simulink model "AthenaSim_2"  (R2024b)
settings: Solver=ode4  StartTime=0.0  StopTime=inf  FixedStep=0.001  RelTol=1e-3
undefined symbols (not defined in the file or in its folder): Payload
libraries: uavmavlinklib x4, dspnetwork x2, shared6dof x1
settings Model: Creator=ercu  LastModifiedBy=ercu

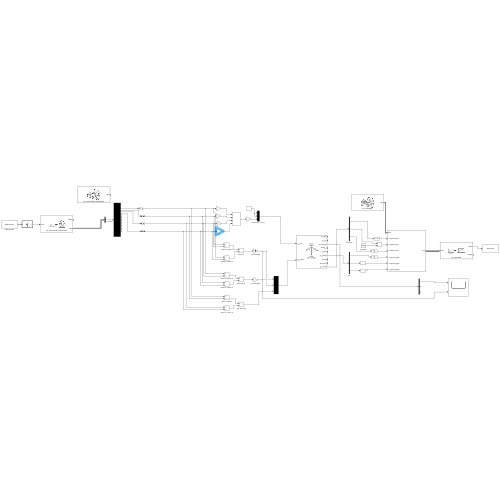
[thumbnail: Simulink's stored preview of the top-level diagram]
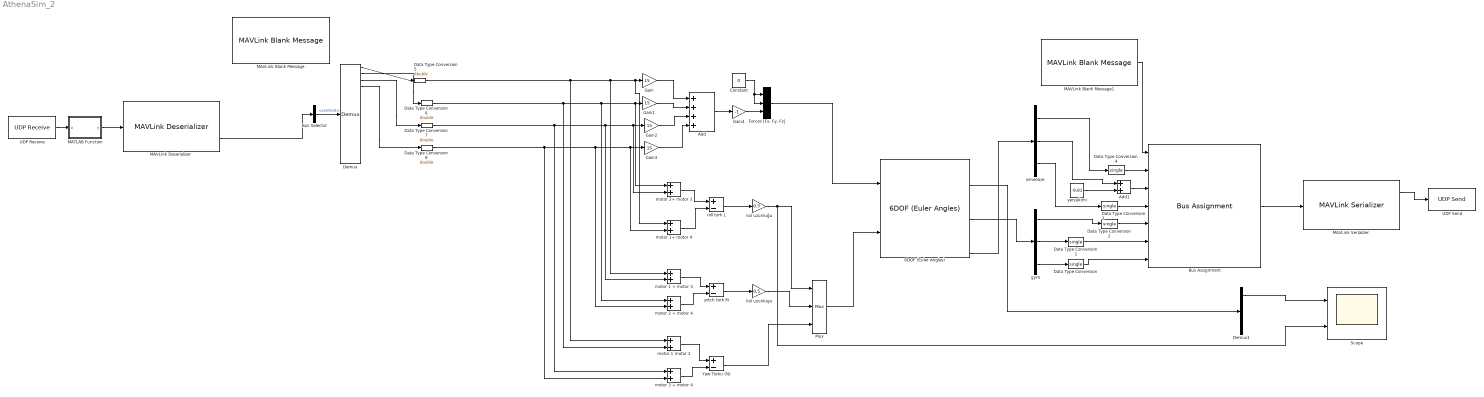
== system AthenaSim_2 ==
  6DOF (Euler Angles) : shared6dof/6DOF (Euler Angles)  units=Metric (MKS)  mtype=Fixed  rep=Euler Angles  xme_0=[0 0 0]  Vm_0=[0 0 0]  eul_0=[0.5 0 0]  pm_0=[0 0 0]  mass_0=1.0  mass_e=0.5  mass_f=2.0  inertia=eye(3) * 0.08  inertia_e=eye(3)  inertia_f=2*eye(3)  k_quat=1.0  vre_flag=on  abi_flag=on  aMode=0  xme_statename=''  Vm_statename=''  eul_statename=''  quat_statename=''  pm_statename=''  mass_statename=''
  Add : Sum  Inputs=++++  OutDataTypeStr=double
  Add1 : Sum  OutDataTypeStr=single
  Bus Assignment : BusAssignment  AssignedSignals=Payload.xacc,Payload.yacc,Payload.zacc,Payload.xgyro,Payload.ygyro,Payload.zgyro
  Bus Selector : BusSelector  OutputSignals=Payload.controls
  Constant : Constant  Value=0
  Data Type Conversion{,1..4} (5 alike) : DataTypeConversion  OutDataTypeStr=single  SaturateOnIntegerOverflow=off  RndMeth=Floor
  Data Type Conversion{5..8} (4 alike) : DataTypeConversion  OutDataTypeStr=double  SaturateOnIntegerOverflow=off  RndMeth=Floor
  Demux : Demux  Outputs=16
  Demux1 : Demux  Outputs=3
  "Forces [Fx, Fy, Fz]" : Mux  Inputs=3
  Gain{,1..3} (4 alike) : Gain  Gain=15
  Gain4 : Gain  Gain=-1
  MATLAB Function : MATLAB Function  TreatAsAtomicUnit=on
  MAVLink Blank Message : uavmavlinklib/MAVLink Blank Message  dialectSource=Select from standard MAVLink dialects  dialect=common.xml  dialectCustom=common.xml  version=2  messageType=HIL_ACTUATOR_CONTROLS  SystemID=1  ComponentID=1  SampleTime=inf
  MAVLink Blank Message1 : uavmavlinklib/MAVLink Blank Message  dialectSource=Select from standard MAVLink dialects  dialect=common.xml  dialectCustom=common.xml  version=2  messageType=HIL_SENSOR  SystemID=1  ComponentID=1  SampleTime=inf
  MAVLink Deserializer : uavmavlinklib/MAVLink Deserializer  dialectSource=Select from standard MAVLink dialects  dialect=common.xml  dialectCustom=common.xml  version=2  messageType=HIL_ACTUATOR_CONTROLS  inputDataLength=off  SystemIDFilter=off  systemID=1  ComponentIDFilter=off  componentID=1  queueMsg=off  queueMsgSize=50  dropNum=off
  MAVLink Serializer : uavmavlinklib/MAVLink Serializer  dialectSource=Select from standard MAVLink dialects  dialect=common.xml  dialectCustom=common.xml  version=2  messageType=HIL_SENSOR
  Mux : Mux  Inputs=3
  Scope : Scope  NumInputPorts=2
  UDP Receive : dspnetwork/UDP Receive  localURL='0.0.0.0'  localPort=14550  remoteURL='127.0.0.1'  remotePort=-1  recvBufferSize=8192  dims=300  signalDatatype=uint8  isComplex=off  isVarSize=on  showBlockingTime=off  blockingTime=0  sampletime=0.001  blockPlatform=[]
      settings: LibrarySourceBlock=dspsrcs4/UDP Receive
  UDP Send : dspnetwork/UDP Send  remoteURL='127.0.0.1'  remotePort=14551  localURL='0.0.0.0'  localPortSource=Automatically determine  localPort=-1  sendBufferSize=8192  sampletime=-1  blockPlatform=[]  separateLengthPort=0
      settings: LibrarySourceBlock=dspsnks4/UDP Send
  Yaw Torku (N) : Sum  Inputs=+-  OutDataTypeStr=double
  gyro : Demux  Outputs=3
  ivmeölçer : Demux  Outputs=3
  kol uzunlugu : Gain  Gain=0.5
  kol uzunluğu : Gain  Gain=0.5
  motor 1 + motor 3 : Sum
  motor 1 motor 2 : Sum
  motor 1+ motor 4 : Sum
  motor 2 + motor 4 : Sum
  motor 2+ motor 3 : Sum
  motor 3 + motor 4 : Sum
  pitch tork M : Sum  Inputs=+-  OutDataTypeStr=double
  roll tork L : Sum  Inputs=+-  OutDataTypeStr=double
  yerçekimi : Constant  Value=-9.81
  wires:
  UDP Receive/1 -> MATLAB Function/1(u)
  MAVLink Deserializer/2 -> Bus Selector/1
  Bus Selector/1 -> Demux/1  "<controls>"
  Demux/1 -> Data Type Conversion5/1
  Demux/2 -> Data Type Conversion6/1
  Demux/3 -> Data Type Conversion7/1
  Demux/4 -> Data Type Conversion8/1
  Data Type Conversion8/1 -> motor 3 + motor 4/2, motor 2 + motor 4/2, motor 1+ motor 4/2, Gain3/1
  Data Type Conversion7/1 -> motor 3 + motor 4/1, motor 1 + motor 3/2, motor 2+ motor 3/2, Gain2/1
  Data Type Conversion6/1 -> motor 1 motor 2/2, motor 2 + motor 4/1, motor 2+ motor 3/1, Gain1/1
  Data Type Conversion5/1 -> motor 1 motor 2/1, motor 1 + motor 3/1, motor 1+ motor 4/1, Gain/1
  Gain/1 -> Add/1
  Gain1/1 -> Add/2
  Gain2/1 -> Add/3
  Gain3/1 -> Add/4
  Add/1 -> Gain4/1
  Gain4/1 -> "Forces [Fx, Fy, Fz]"/3
  Constant/1 -> "Forces [Fx, Fy, Fz]"/1, "Forces [Fx, Fy, Fz]"/2
  motor 2+ motor 3/1 -> roll tork L/1
  motor 1+ motor 4/1 -> roll tork L/2
  roll tork L/1 -> kol uzunluğu/1
  pitch tork M/1 -> kol uzunlugu/1
  motor 1 + motor 3/1 -> pitch tork M/1
  motor 2 + motor 4/1 -> pitch tork M/2
  motor 1 motor 2/1 -> Yaw Torku (N)/1
  motor 3 + motor 4/1 -> Yaw Torku (N)/2
  kol uzunluğu/1 -> Scope/2, Mux/1
  kol uzunlugu/1 -> Mux/2
  Yaw Torku (N)/1 -> Mux/3
  "Forces [Fx, Fy, Fz]"/1 -> 6DOF (Euler Angles)/1
  Mux/1 -> 6DOF (Euler Angles)/2
  MAVLink Serializer/1 -> UDP Send/1
  6DOF (Euler Angles)/6 -> gyro/1
  6DOF (Euler Angles)/9 -> ivmeölçer/1
  MAVLink Blank Message1/1 -> Bus Assignment/1
  ivmeölçer/1 -> Data Type Conversion4/1
  ivmeölçer/2 -> Add1/1
  ivmeölçer/3 -> Data Type Conversion3/1
  gyro/1 -> Data Type Conversion2/1
  gyro/2 -> Data Type Conversion1/1
  gyro/3 -> Data Type Conversion/1
  Bus Assignment/1 -> MAVLink Serializer/1
  yerçekimi/1 -> Add1/2
  Add1/1 -> Bus Assignment/3
  6DOF (Euler Angles)/3 -> Demux1/1
  Demux1/1 -> Scope/1
  Data Type Conversion/1 -> Bus Assignment/7
  Data Type Conversion1/1 -> Bus Assignment/6
  Data Type Conversion2/1 -> Bus Assignment/5
  Data Type Conversion3/1 -> Bus Assignment/4
  Data Type Conversion4/1 -> Bus Assignment/2
  MATLAB Function/1(y) -> MAVLink Deserializer/1

== matlab function AthenaSim_2/MATLAB Function ==
  data: u input; y output
function y = fix_data(u)
    % Girişin boyutunu ve tipini ayarla
    % UDP'den ne gelirse gelsin, çıkış her zaman 300 elemanlı uint8 dizisi olsun.
    
    % Sabit boyutlu bir sıfır dizisi oluştur
    y = zeros(300, 1, 'uint8');
    
    % Eğer gelen veri boş değilse, y'nin içine kopyala
    if ~isempty(u)
        len = min(length(u), 300);
        y(1:len) = u(1:len);
    end
end
